simulink model "PMSM_Relay3_inverter"  (R2022b)
settings: Solver=ode23tb  StartTime=0.0  StopTime=0.1  RelTol=1e-4
libraries: spsUniversalBridgeLib x1, spsPermanentMagnetSynchronousMachineLib x1, spsDCVoltageSourceLib x1, sps_lib x1
Description:
  | Copyright 2008-2014 The MathWorks, Inc.
settings Model: Creator=MathWorks  LastModifiedBy=Guoguo
settings SolverCC: AlgebraicLoopSolver=TrustRegion
settings DataIOCC: ExternalInput=[]  SaveFormat=Array  SignalLoggingSaveFormat=ModelDataLogs  SaveOutput=off  SaveTime=off  ReturnWorkspaceOutputs=off  SignalLoggingName=sigsOut
settings OptimizationCC: BlockReduction=off  BooleanDataType=off  ExpressionDepthLimit=2147483647  InitFltsAndDblsToZero=on  EfficientMapNaN2IntZero=off  LifeSpan=inf
settings DebuggingCC: UnderspecifiedInitializationDetection=Classic  MergeDetectMultiDrivingBlocksExec=none  CheckExecutionContextPreStartOutputMsg=on  SignalResolutionControl=TryResolveAllWithWarning  MultiTaskDSMMsg=warning  MultiTaskCondExecSysMsg=none  SigSpecEnsureSampleTimeMsg=none  FcnCallInpInsideContextMsg=warning  UnconnectedInputMsg=warning  UnconnectedOutputMsg=warning  UnconnectedLineMsg=warning  StateNameClashWarn=warning  SFUnexpectedBacktrackingDiag=warning  SFNoUnconditionalDefaultTransitionDiag=warning  SFExecutionAtInitializationDiag=none  SFMachineParentedDataDiag=warning  ArithmeticOperatorsInVariantConditions=warning
settings HardwareCC: ProdBitPerPointer=32  ProdBitPerSizeT=32  ProdBitPerPtrDiffT=32  ProdLargestAtomicFloat=None  ProdIntDivRoundTo=Undefined  ProdEndianess=Unspecified  ProdWordSize=32  ProdHWDeviceType=32-bit Generic  TargetUnknown=on
settings ModelReferenceCC: EnableRefExpFcnMdlSchedulingChecks=on  PropagateSignalLabelsOutOfModel=off
settings SFSimCC: SimUseLocalCustomCode=off  CustomCodeUndefinedFunction=UseInterfaceOnly
settings RTWCC: RTWUseLocalCustomCode=off  DLArmComputeVersion=19.05
settings CodeAppCC: StateflowObjectComments=on
settings GRTTargetCC: TargetLangStandard=C89/C90 (ANSI)  CombineOutputUpdateFcns=off  GRTInterface=on
settings ConfigComp: CovMetricSettings=dw  CovSaveCumulativeToWorkspaceVar=on  CovSaveSingleToWorkspaceVar=on  CovExternalEMLEnable=off  CovSFcnEnable=off
settings SimscapeCC: SimscapeNormalizeSystem=off

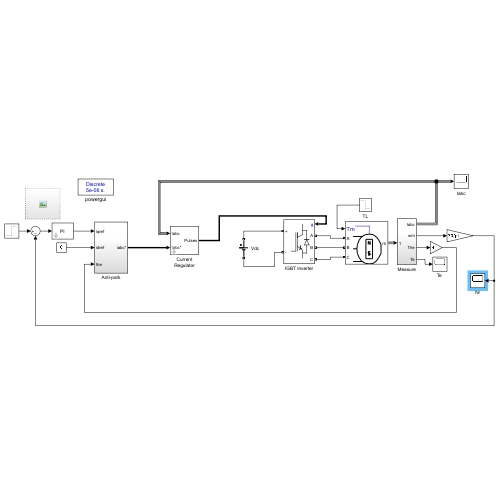
[thumbnail: Simulink's stored preview of the top-level diagram]
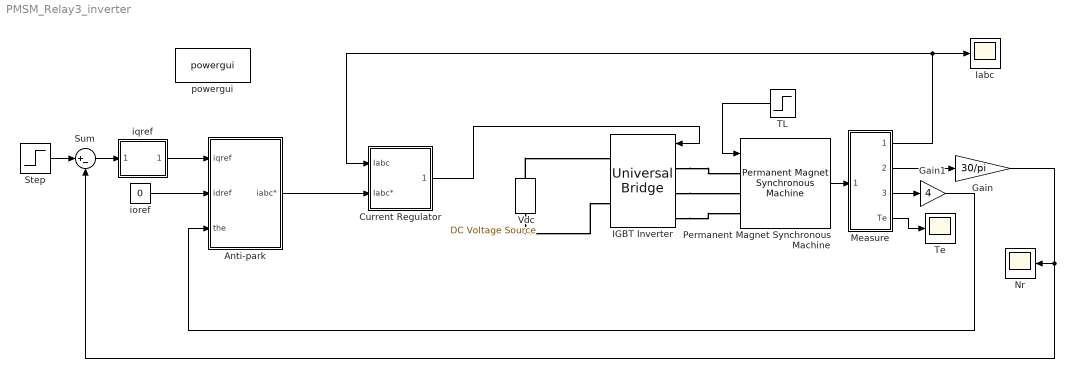
== system PMSM_Relay3_inverter ==
  Anti-park : Subsystem
  Current Regulator : Subsystem  mask(Regulateur de courant a hysteresis){h=0.02}
      mask prompts: h "Hysteresis band (A)"
  Gain : Gain  Gain=30/pi  SaturateOnIntegerOverflow=on  OutDataTypeStr=Inherit: Same as input  ParamDataTypeStr=Inherit: Same as input
  Gain1 : Gain  Gain=4  SaturateOnIntegerOverflow=on  OutDataTypeStr=Inherit: Same as input  ParamDataTypeStr=Inherit: Same as input
  IGBT Inverter : spsUniversalBridgeLib/Universal Bridge  Arms=3  SnubberResistance=1000  SnubberCapacitance=inf  Device=IGBT / Diodes  Ron=1e-3  Lon=0  ForwardVoltages="[  0.8  0.8  ]"  ForwardVoltage=.8  GTOparameters=[ 1e-6 , 1e-6 ]  IGBTparameters=[ 1e-6 , 2e-6 ]  Measurements=None  Measurements_2=None  converterType=Rectifier
      settings: AttributesFormatString=\n
  Iabc : Scope
  Measure : Subsystem
  Nr : Scope
  Permanent Magnet Synchronous Machine : spsPermanentMagnetSynchronousMachineLib/Permanent Magnet Synchronous Machine  NbPhases=3  FluxDistribution=Sinusoidal  RotorType=Salient-pole  MechanicalLoad=Torque Tm  PresetModel=No  ShowDetailedParameters=on  MeasurementBus=off  Resistance=2.875  Inductance=8.5e-3  dqInductances=[8.5e-3,8.5e-3]  La=0.00153  MachineConstant=Flux linkage established by magnets (V.s)  Flux=0.175  VoltageCst=126.966  TorqueCst=1.05  Flat=120  Mechanical=[0.8e-3, 0 4]  PolePairs=4  InitialConditions=[0,0, 0,0]  InitialConditions5ph=[0 0 0 0 0 0]  RefAngle=Aligned with phase A axis (original Park)  IterativeDiscreteModel=Trapezoidal non iterative  TsBlock=-1  TsPowergui=0
  Step : Step  Time=0.05  Before=800  After=1500  SampleTime=0
  Sum : Sum  Inputs=|+-
  TL : Step  Time=0.05  Before=3  SampleTime=0
  "Te " : Scope
  Vdc : spsDCVoltageSourceLib/DC Voltage Source  Description=source block  Amplitude=780  Measurements=None
      settings: AttributesFormatString=\n
  ioref : Constant  Value=0
  iqref : Subsystem  mask(PI Controller){I=0.06, P=1, sat=[-30, 30]}
      mask prompts: I "Integral"; P "Proportional:"; sat "Minimum and maximum outputs:"
      mask init:
      | min=sat(1);max=sat(2);
      mask Display: disp('PI')
  powergui : sps_lib/powergui  SimulationMode=Discrete  SampleTime=5e-6  frequency=60  Iterations=50  frequencyindice=0  Pbase=100e6  ErrMax=1e-4  UnitsV=kV  UnitsW=MW  buscounter=0  FunctionMessages=off  echomessages=off  EnableUseOfTLC=off  CurrentSourceSwitches=off  DisableSnubberDevices=off  DisableRonSwitches=off  DisableVfSwitches=off  DisplayEquations=off  AutomaticDiscreteSolvers=off  SolverType=Tustin  Interpol=off  ExternalGateDelay=off  methode=off  Ts=0  x0status=blocks  SPID=on  SwTol=0  HookPort=off  NonlinearTolerance=1e-4  nMaxIteration=100  ContinueOnMaxIteration=off  RestoreLinks=warning  ResistiveCurrentMeasurement=off  Frange=[0:2:500]  Ylog=off  Xlog=on  ShowGrid=off  save=off  variable=ZData  structure=0  ZoomFFT=on  StartTime=0.0  cycles=1  DisplayStyle=1  fundamental=60  FreqAxis=off  MaxFrequency=1000  frequencyindicesteady=1  RmsSteady=1  display=off
  wires:
  ioref/1 -> Anti-park/2(idref)
  Sum/1 -> iqref/1(In_1)
  Step/1 -> Sum/1
  iqref/1(Out_1) -> Anti-park/1(iqref)
  Gain/1 -> Nr/1, Sum/2
  TL/1 -> Permanent Magnet Synchronous Machine/1
  Measure/1(Iabc) -> Current Regulator/1(Iabc), Iabc/1
  Permanent Magnet Synchronous Machine/1 -> Measure/1(In1)
  Measure/2(wm) -> Gain/1
  Measure/3(The) -> Gain1/1
  Measure/4(Te) -> "Te "/1
  Gain1/1 -> Anti-park/3(the)
  Current Regulator/1(Pulses) -> IGBT Inverter/1
  Anti-park/1(iabc*) -> Current Regulator/2(Iabc*)
  connections:
  Vdc/RConn1 -- IGBT Inverter/RConn1
  Vdc/LConn1 -- IGBT Inverter/RConn2
  IGBT Inverter/LConn2 -- Permanent Magnet Synchronous Machine/LConn2
  IGBT Inverter/LConn1 -- Permanent Magnet Synchronous Machine/LConn1
  IGBT Inverter/LConn3 -- Permanent Magnet Synchronous Machine/LConn3

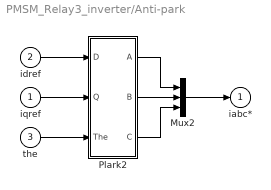
== system PMSM_Relay3_inverter/Anti-park ==
  iqref : Inport
  idref : Inport  Port=2
  the : Inport  Port=3
  Mux2 : Mux  Inputs=3
  Plark2 : Subsystem
  iabc* : Outport  InitialOutput=0
  wires:
  the/1 -> Plark2/3(The)
  idref/1 -> Plark2/1(D)
  iqref/1 -> Plark2/2(Q)
  Plark2/2(B) -> Mux2/2
  Plark2/1(A) -> Mux2/1
  Plark2/3(C) -> Mux2/3
  Mux2/1 -> iabc*/1

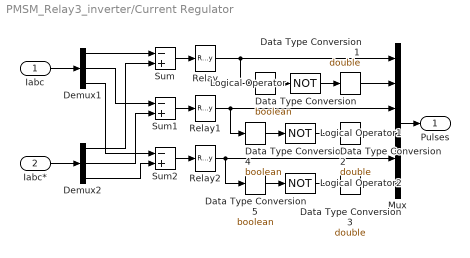
== system PMSM_Relay3_inverter/Current Regulator ==
  Iabc : Inport
  Iabc* : Inport  Port=2
  Data Type Conversion : DataTypeConversion  OutDataTypeStr=boolean
  Data Type Conversion1 : DataTypeConversion  OutDataTypeStr=double
  Data Type Conversion2 : DataTypeConversion  OutDataTypeStr=double
  Data Type Conversion3 : DataTypeConversion  OutDataTypeStr=double
  Data Type Conversion4 : DataTypeConversion  OutDataTypeStr=boolean
  Data Type Conversion5 : DataTypeConversion  OutDataTypeStr=boolean
  Demux1 : Demux  Outputs=3
      settings: DisplayOption=none
  Demux2 : Demux  Outputs=3
      settings: DisplayOption=none
  Logical Operator : Logic  Operator=NOT
  Logical Operator1 : Logic  Operator=NOT
  Logical Operator2 : Logic  Operator=NOT
  Mux : Mux  Inputs=6
  Relay : Relay  OnSwitchValue=h/2  OffSwitchValue=-h/2
  Relay1 : Relay  OnSwitchValue=h/2  OffSwitchValue=-h/2
  Relay2 : Relay  OnSwitchValue=h/2  OffSwitchValue=-h/2
  Sum : Sum  Inputs=-+  InputSameDT=on  SaturateOnIntegerOverflow=on  OutDataTypeStr=Inherit: Same as first input
  Sum1 : Sum  Inputs=-+  InputSameDT=on  SaturateOnIntegerOverflow=on  OutDataTypeStr=Inherit: Same as first input
  Sum2 : Sum  Inputs=-+  InputSameDT=on  SaturateOnIntegerOverflow=on  OutDataTypeStr=Inherit: Same as first input
  Pulses : Outport  InitialOutput=0
  wires:
  Sum/1 -> Relay/1
  Sum1/1 -> Relay1/1
  Demux1/1 -> Sum/1
  Demux1/2 -> Sum1/1
  Mux/1 -> Pulses/1
  Iabc/1 -> Demux1/1
  Sum2/1 -> Relay2/1
  Demux1/3 -> Sum2/1
  Demux2/3 -> Sum2/2
  Demux2/2 -> Sum1/2
  Demux2/1 -> Sum/2
  Iabc*/1 -> Demux2/1
  Relay/1 -> Mux/1, Data Type Conversion/1
  Relay1/1 -> Mux/3, Data Type Conversion4/1
  Relay2/1 -> Mux/5, Data Type Conversion5/1
  Data Type Conversion/1 -> Logical Operator/1
  Logical Operator/1 -> Data Type Conversion1/1
  Data Type Conversion1/1 -> Mux/2
  Logical Operator1/1 -> Data Type Conversion2/1
  Data Type Conversion2/1 -> Mux/4
  Logical Operator2/1 -> Data Type Conversion3/1
  Data Type Conversion3/1 -> Mux/6
  Data Type Conversion4/1 -> Logical Operator1/1
  Data Type Conversion5/1 -> Logical Operator2/1

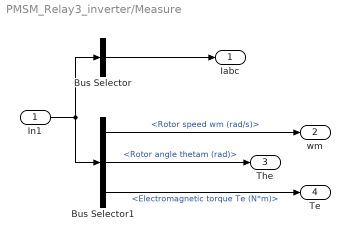
== system PMSM_Relay3_inverter/Measure ==
  In1 : Inport
  Bus Selector : BusSelector  OutputSignals=Stator current is_a (A),Stator current is_b (A),Stator current is_c (A)  OutputAsBus=on
  Bus Selector1 : BusSelector  OutputSignals=Rotor speed wm (rad/s),Rotor angle thetam (rad),Electromagnetic torque Te (N*m)
  Iabc : Outport
  wm : Outport  Port=2
  The : Outport  Port=3
  Te : Outport  Port=4
  wires:
  Bus Selector1/1 -> wm/1  "<Rotor speed wm (rad/s)>"
  Bus Selector1/2 -> The/1  "<Rotor angle thetam (rad)>"
  Bus Selector/1 -> Iabc/1
  Bus Selector1/3 -> Te/1  "<Electromagnetic torque Te (N*m)>"
  In1/1 -> Bus Selector1/1, Bus Selector/1

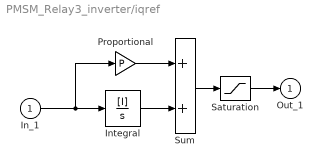
== system PMSM_Relay3_inverter/iqref ==
  In_1 : Inport
  Integral : TransferFcn  Numerator=[I]  Denominator=[1 0]
  Proportional : Gain  Gain=P  SaturateOnIntegerOverflow=on  OutDataTypeStr=Inherit: Same as input  ParamDataTypeStr=Inherit: Same as input
  Saturation : Saturate  UpperLimit=max  LowerLimit=min
  Sum : Sum  InputSameDT=on  SaturateOnIntegerOverflow=on  OutDataTypeStr=Inherit: Same as first input
  Out_1 : Outport  InitialOutput=0
  wires:
  Integral/1 -> Sum/2
  In_1/1 -> Integral/1, Proportional/1
  Proportional/1 -> Sum/1
  Sum/1 -> Saturation/1
  Saturation/1 -> Out_1/1

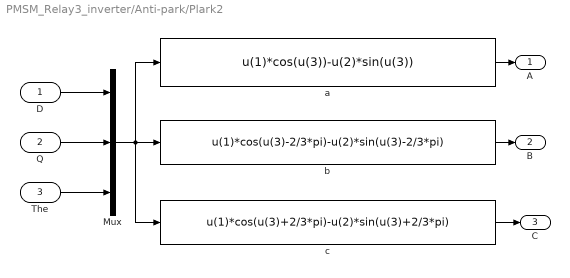
== system PMSM_Relay3_inverter/Anti-park/Plark2 ==
  D : Inport
  Q : Inport  Port=2
  The : Inport  Port=3
  Mux : Mux  Inputs=3
  a : Fcn  Expr=u(1)*cos(u(3))-u(2)*sin(u(3))
  b : Fcn  Expr=u(1)*cos(u(3)-2/3*pi)-u(2)*sin(u(3)-2/3*pi)
  c : Fcn  Expr=u(1)*cos(u(3)+2/3*pi)-u(2)*sin(u(3)+2/3*pi)
  A : Outport
  B : Outport  Port=2
  C : Outport  Port=3
  wires:
  b/1 -> B/1
  The/1 -> Mux/3
  a/1 -> A/1
  D/1 -> Mux/1
  Q/1 -> Mux/2
  Mux/1 -> c/1, a/1, b/1
  c/1 -> C/1
